simulink model "simple_test"  (R2015b)
settings: Solver=VariableStepAuto  StartTime=0.0  StopTime=inf  RelTol=1e-3
values from neighbouring files (symbols this model uses):
  P = 4    [BLDCmotor_modeling_param.m]
undefined symbols (not defined in the file or in its folder): trapezoid
libraries: aerolibanimutils x1
settings Model: Creator=shangwei  LastModifiedBy=root

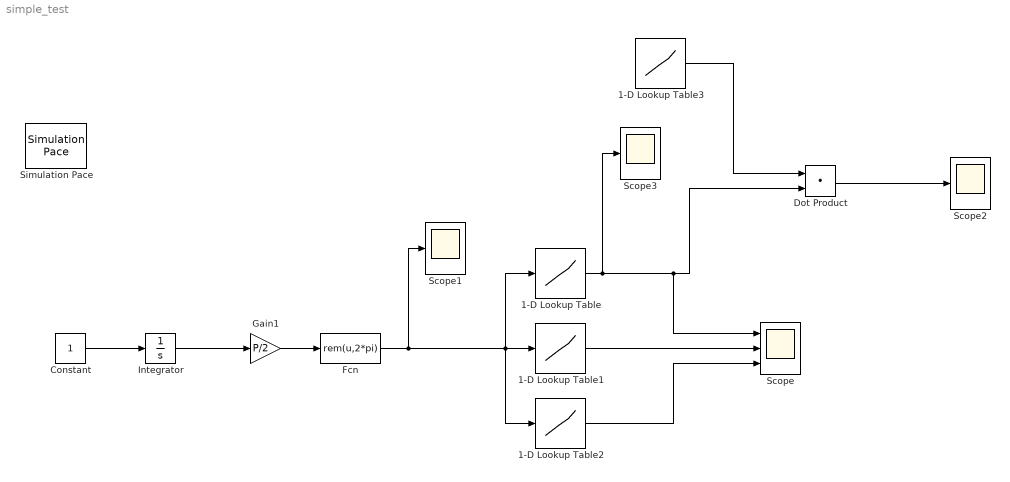
== system simple_test ==
  1-D Lookup Table : Lookup_n-D  NumberOfTableDimensions=1  BreakpointsForDimension1=0:0.001:2*pi  Table=trapezoid(0:0.001:2*pi,0)  InternalRulePriority=Speed  RndMeth=Simplest  InputSameDT=on
  1-D Lookup Table1 : Lookup_n-D  NumberOfTableDimensions=1  BreakpointsForDimension1=((0:0.001:2*pi))  Table=trapezoid(0:0.001:2*pi, 2/3*pi)  InternalRulePriority=Speed  RndMeth=Simplest  InputSameDT=on
  1-D Lookup Table2 : Lookup_n-D  NumberOfTableDimensions=1  BreakpointsForDimension1=(0:0.001:2*pi)  Table=trapezoid(0:0.001:2*pi, 4/3*pi)  InternalRulePriority=Speed  RndMeth=Simplest  InputSameDT=on
  1-D Lookup Table3 : Lookup_n-D  NumberOfTableDimensions=1  BreakpointsForDimension1=0:0.001:2*pi  Table=trapezoid(0:0.001:2*pi,0)  InternalRulePriority=Speed  RndMeth=Simplest  InputSameDT=on
  Constant : Constant
  Dot Product : DotProduct  InputSameDT=on  OutDataTypeStr=Inherit: Inherit via internal rule
  Fcn : Fcn  Expr=rem(u,2*pi)
  Gain1 : Gain  Gain=P/2
  Integrator : Integrator
  Scope : Scope  NumInputPorts=3
  Scope1 : Scope
  Scope2 : Scope
  Scope3 : Scope
  Simulation Pace : aerolibanimutils/Simulation Pace  SimulationPace=1  SleepMode=MATLAB Thread  OutputPaceError=off  SampleTime=1/30
  wires:
  Fcn/1 -> Scope1/1, 1-D Lookup Table2/1, 1-D Lookup Table1/1, 1-D Lookup Table/1
  1-D Lookup Table/1 -> Scope3/1, Scope/1, Dot Product/2
  1-D Lookup Table1/1 -> Scope/2
  1-D Lookup Table2/1 -> Scope/3
  Gain1/1 -> Fcn/1
  Integrator/1 -> Gain1/1
  Constant/1 -> Integrator/1
  Dot Product/1 -> Scope2/1
  1-D Lookup Table3/1 -> Dot Product/1
